simulink model "zadatak4"  (R2024a)
settings: Solver=ode23t  StartTime=0.0  StopTime=5  RelTol=1e-3
PreLoadFcn:
  | mdl_puma560
libraries: roblocks x4
settings Model: Creator=Mirza
settings ModelReferenceCC: EnableRefExpFcnMdlSchedulingChecks=on
settings RTWCC: GPUComputeCapability=3.5

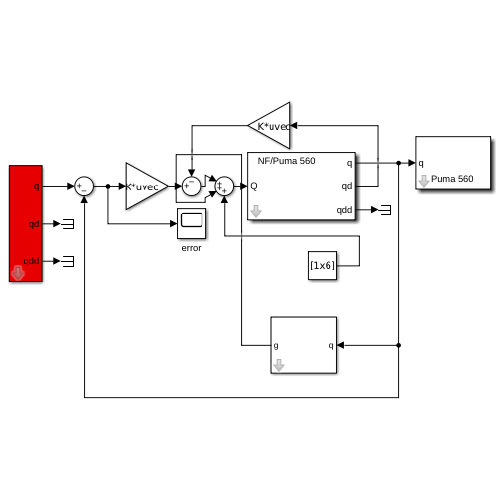
[thumbnail: Simulink's stored preview of the top-level diagram]
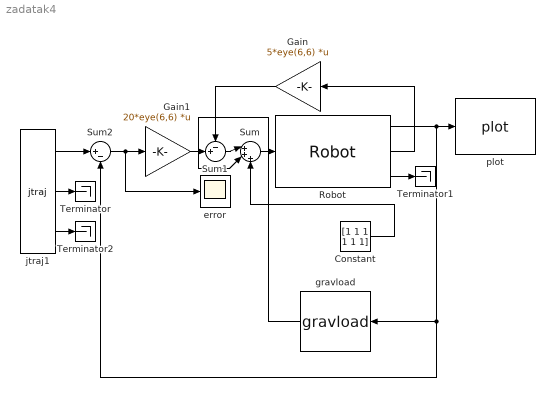
== system zadatak4 ==
  Constant : Constant  Value=[1 1 1 1 1 1]
  Gain : Gain  Gain=5*eye(6,6)  Multiplication=Matrix(K*u) (u vector)
  Gain1 : Gain  Gain=20*eye(6,6)  Multiplication=Matrix(K*u) (u vector)
  Robot : roblocks/Arm/Robot  robot=p560.nofriction  q0=[0 0 0 0 0 0]
  Sum : Sum  Inputs=|+++
  Sum1 : Sum  Inputs=-+|
  Sum2 : Sum  Inputs=|+-
  Terminator : Terminator
  Terminator1 : Terminator
  Terminator2 : Terminator
  error : Scope
  gravload : roblocks/Arm/gravload  robot=p560.nofriction
  jtraj1 : roblocks/Toolbox/jtraj  q0=[0 0 0 0 0 0]  qf=[0 0 0 pi/2 pi/4 pi/3 ]  tmax=3  ts=0
  plot : roblocks/Arm/plot  robot=p560  fps=25  holdplot=on
  wires:
  jtraj1/2 -> Terminator/1
  jtraj1/1 -> Sum2/1
  Sum1/1 -> Sum/1
  Robot/1 -> plot/1, Sum2/2, gravload/1
  gravload/1 -> Sum/2
  Robot/3 -> Terminator1/1
  Robot/2 -> Gain/1
  Gain/1 -> Sum1/1
  Gain1/1 -> Sum1/2
  Sum2/1 -> error/1, Gain1/1
  Sum/1 -> Robot/1
  jtraj1/3 -> Terminator2/1
  Constant/1 -> Sum/3
